simulink model "triggeredsub"  (R2019b)
settings: Solver=VariableStepDiscrete  StartTime=0.0  StopTime=8  MaxStep=.1  RelTol=1e-3  EnableMultiTasking=on
Description:
  | Triggered Subsystems
  | 
  | This model shows triggered subsystems and describes the different trigger types. A
  | triggered subsystem is executed for a single time step whenever the trigger port
  | transitions from false to true in a specified direction. The transition of the trigger port
  | may occur when the direction of the transition is rising, falling, or both rising and
  | falling. A rising transition occurs when the trigger signal transitions from zero or
  | below to a positive value. A falling transition occurs when the trigger signal transitions
  | from zero or above to a negative value.
  | 
  | After running the simulation, look closely at the top plot in the scope. This shows a sine
  | wave, a waveform, and the grounded value of zero. As the waveform transitions
  | through zero, each of the subsystems is triggered appropriately. The output of each
  | subsystem is equal to the current value of the sine wave at that time.
settings Model: ExtModeTrigMode=oneshot  ExtModeArmWhenConnect=off  ExtModeAutoUpdateStatusClock=off  Creator=The MathWorks, Inc.  LastModifiedBy=bhisma
settings DataIOCC: SaveFormat=Array
settings OptimizationCC: BlockReduction=off  BooleanDataType=off  ExpressionDepthLimit=2147483647  InitFltsAndDblsToZero=on  LifeSpan=inf  BufferReusableBoundary=off
settings DebuggingCC: SaveWithParameterizedLinksMsg=none  SignalResolutionControl=TryResolveAllWithWarning  MultiTaskDSMMsg=warning  MultiTaskCondExecSysMsg=none  IntegerOverflowMsg=none  FcnCallInpInsideContextMsg=warning  BusObjectLabelMismatch=none  AllowSymbolicDim=off  StateNameClashWarn=warning  SFUnexpectedBacktrackingDiag=warning  SFNoUnconditionalDefaultTransitionDiag=warning  SFExecutionAtInitializationDiag=none  IntegerSaturationMsg=none  ArithmeticOperatorsInVariantConditions=warning
settings HardwareCC: ProdBitPerPointer=32  ProdBitPerSizeT=32  ProdBitPerPtrDiffT=32  ProdLargestAtomicFloat=None  ProdIntDivRoundTo=Undefined  ProdEndianess=Unspecified  ProdWordSize=32  ProdHWDeviceType=32-bit Generic  TargetUnknown=on
settings ModelReferenceCC: PropagateSignalLabelsOutOfModel=off
settings SFSimCC: SimUseLocalCustomCode=off  CustomCodeUndefinedFunction=UseInterfaceOnly
settings RTWCC: Description=Generic Real-Time Target  RTWUseLocalCustomCode=off
settings CodeAppCC: StateflowObjectComments=on
settings GRTTargetCC: TargetFcnLib=ansi_tfl_tmw.mat  TargetLangStandard=C89/C90 (ANSI)  GeneratePreprocessorConditionals=Disable all  CombineOutputUpdateFcns=off  GRTInterface=on
settings ConfigComp: CovMetricSettings=dw  CovHtmlReporting=on  CovSaveCumulativeToWorkspaceVar=on  CovSaveSingleToWorkspaceVar=on  CovExternalEMLEnable=off  CovSFcnEnable=off

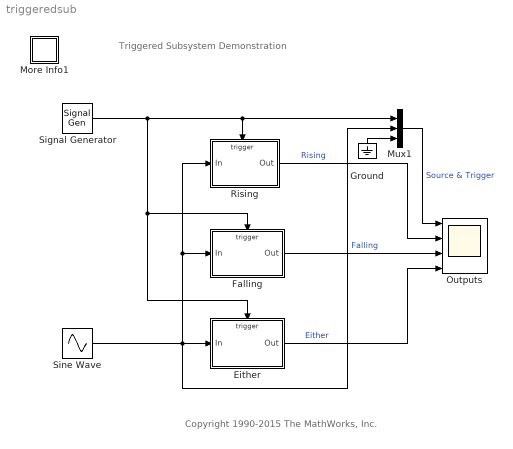
== system triggeredsub ==
  note: Triggered Subsystem Demonstration
  note: Copyright 1990-2015 The MathWorks, Inc.
  Either : Subsystem
  Falling : Subsystem
  Ground : Ground
  More Info1 : Subsystem
      settings: OpenFcn=showdemo(bdroot(gcs))
      mask Display: disp('?')
  Mux1 : Mux  Inputs=3
  Outputs : Scope  NumInputPorts=4
      settings: StartFcn=open_system(gcbh)
  Rising : Subsystem
  Signal Generator : SignalGenerator  WaveForm=square  Amplitude=0.5
      settings: AttributesFormatString=Waveform: %<waveform>\nFreq: %<Frequency> %<Units>
  Sine Wave : Sin  Frequency=8  SampleTime=0
      settings: AttributesFormatString=Freq: %<Frequency> rad/sec
  wires:
  Signal Generator/1 -> Rising/Trigger, Mux1/1, Either/Trigger, Falling/Trigger
  Sine Wave/1 -> Falling/1(In), Rising/1(In), Either/1(In), Mux1/2
  Ground/1 -> Mux1/3
  Rising/1(Out) -> Outputs/2  "Rising"
  Falling/1(Out) -> Outputs/3  "Falling"
  Either/1(Out) -> Outputs/4  "Either"
  Mux1/1 -> Outputs/1  "Source & Trigger"

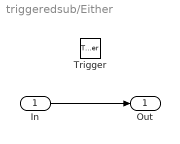
== system triggeredsub/Either ==
  In : Inport
  Trigger : TriggerPort  TriggerType=either  VariantControl=(inherit)
  Out : Outport  InitialOutput=0  VectorParamsAs1DForOutWhenUnconnected=off
  wires:
  In/1 -> Out/1

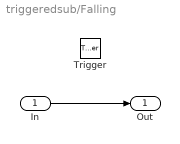
== system triggeredsub/Falling ==
  In : Inport
  Trigger : TriggerPort  TriggerType=falling  VariantControl=(inherit)
  Out : Outport  InitialOutput=0  VectorParamsAs1DForOutWhenUnconnected=off
  wires:
  In/1 -> Out/1

== system triggeredsub/More Info1 ==

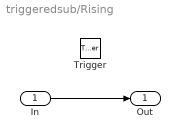
== system triggeredsub/Rising ==
  In : Inport
  Trigger : TriggerPort  VariantControl=(inherit)
  Out : Outport  InitialOutput=0  VectorParamsAs1DForOutWhenUnconnected=off
  wires:
  In/1 -> Out/1
